simulink model "simulation1"  (R2018a)
settings: Solver=FixedStepAuto  StartTime=0.0  StopTime=300  FixedStep=0.1  RelTol=1e-3
values from neighbouring files (symbols this model uses):
  C_wn = C_w(:,4)    [Sim1.m]    (also in Sim3.m; Sim4_EKF.m; Sim4_Nolinear.m; Sim5_Nolinear.m)
  C_wx = C_w(:,2)    [Sim1.m]    (also in Sim3.m; Sim4_EKF.m; Sim4_Nolinear.m; Sim5_Nolinear.m)
  C_wy = C_w(:,3)    [Sim1.m]    (also in Sim3.m; Sim4_EKF.m; Sim4_Nolinear.m; Sim5_Nolinear.m)
  getPos = [0;0;1]    [Sim2.m]    (also in Sim3.m; Sim4_EKF.m; Sim4_Nolinear.m; Sim5_Nolinear.m)
  getVel = [0;1;0]    [Sim2.m]    (also in Sim3.m; Sim4_EKF.m; Sim4_Nolinear.m; Sim5_Nolinear.m)
  h = 0.1    [Sim1.m]    (also in Sim2.m; Sim3.m; Sim4_EKF.m; Sim4_Nolinear.m)
  Kd = 7*[2*M3(1)*Omega 0 0; 0 3*M3(2,2)*Omega 0; 0 0 20*M(3,3)*Omega]    [Sim2.m]    (also in Sim3.m; Sim4_EKF.m; Sim4_Nolinear.m; Sim5_Nolinear.m = 7*[30*M3(1)*Omega 0 0; 0 150*M3(2,2)*Omega 0; 0 0 30*M(3,3)*)
  Ki = 100*(omega/10)*[M3(1)*omega^2 0 0;0 0.05*M3(2,2)*omega^2 0; 0 0 M3(3,3)*omega^2 ]*2    [Sim2.m]    (also in Sim3.m; Sim4_EKF.m; Sim4_Nolinear.m; Sim5_Nolinear.m = 10*(omega/10)*[30*M3(1)*omega^2 0 0;0 150*M3(2,2)*omega^2 0;)
  Kp = 50*[6*M3(1)*omega^2 0 0;0 M3(2,2)*omega^2 0; 0 0 10*M3(3,3)*omega^2 ]    [Sim2.m]    (also in Sim3.m; Sim4_EKF.m; Sim4_Nolinear.m; Sim5_Nolinear.m = 5*[60*M3(1)*omega^2 0 0;0 800*M3(2,2)*omega^2 0; 0 0 30*M3(3)
  mu2_c = 0.001    [Sim1.m]    (also in Sim3.m; Sim4_EKF.m; Sim4_Nolinear.m; Sim5_Nolinear.m)
  mu2_w = 0.001    [Sim1.m]    (also in Sim3.m; Sim4_EKF.m; Sim4_Nolinear.m; Sim5_Nolinear.m)
  mu_w = 0.001    [Sim1.m]    (also in Sim3.m; Sim4_EKF.m; Sim4_Nolinear.m; Sim5_Nolinear.m)
  Omega = 2*damping*omega    [Sim2.m]    (also in Sim3.m; Sim4_EKF.m; Sim4_Nolinear.m = diag([omega_1,omega_2,omega_3]); Sim5_Nolinear.m = diag([omega_1,omega_2,omega_3]))
  omega = omegab/sqrt(1-2*damping^2+sqrt(4*damping^4-4*damping^2+2))    [Sim2.m]    (also in Sim3.m; Sim4_EKF.m; Sim4_Nolinear.m; Sim5_Nolinear.m)
  phi_c = -pi/2    (= -1.57079632679)    [Sim1.m]    (also in Sim3.m; Sim4_EKF.m; Sim4_Nolinear.m; Sim5_Nolinear.m)
  psi_r = C_w(:,1)    [Sim1.m]    (also in Sim3.m; Sim4_EKF.m; Sim4_Nolinear.m; Sim5_Nolinear.m)
  ref = [0;0;0]    [Sim2.m]    (also in Sim3.m; Sim4_EKF.m; Sim4_Nolinear.m; Sim5_Nolinear.m)
  V_mean = 0.5    [Sim1.m]    (also in Sim3.m; Sim4_EKF.m; Sim4_Nolinear.m; Sim5_Nolinear.m)
  W_gust = Ug    [Sim1.m]    (also in Sim3.m; Sim4_EKF.m; Sim4_Nolinear.m; Sim5_Nolinear.m)
  W_mean = 15    [Sim1.m]    (also in Sim3.m; Sim4_EKF.m; Sim4_Nolinear.m; Sim5_Nolinear.m)
undefined symbols (not defined in the file or in its folder): Hoerner, magnitude, vessel
libraries: simulink x3, marine_hydro x2, marine_gnc x1, simulink_extras x1
settings Model: Creator=jonbjor  LastModifiedBy=34275

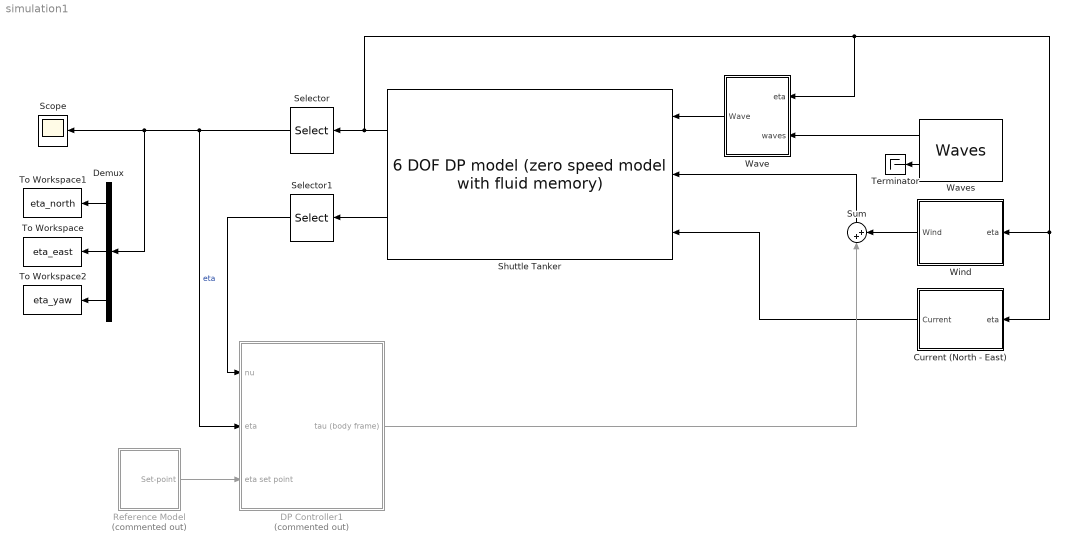
== system simulation1 ==
  Current (North - East) : Subsystem
  DP Controller1 : Subsystem  Commented=on
  Demux : Demux  Outputs=3
  Reference Model : Subsystem  Commented=on
  Scope : Scope
  Selector : Selector  InputPortWidth=6  IndexOptions=Index vector (dialog)  Indices=[1 2 6]  OutputSizes=1
  Selector1 : Selector  InputPortWidth=6  IndexOptions=Index vector (dialog)  Indices=[1 2 6]  OutputSizes=1
  Shuttle Tanker : marine_hydro/Hydro Library/6 DOF DP model  (zero speed model with fluid memory)  ABC=vesselABC  rho=1025  Axc=0.9*vessel.main.T*vessel.main.B  Ayc=0.9*vessel.main.T*vessel.main.Lpp  CX=1  CY_2D=Hoerner(vessel.main.B,vessel.main.T)  Bv=vessel.Bv  mask(6 DOF zero speed model){}
      link override "Integrator1 ": InitialCondition=nu0
      link override Integrator2: InitialCondition=eta0
      settings: SourceProductName=MSS Hydro
      mask Display:
      | image('shuttleTanker.jpg');
      | color('white'); port_label('output', 1, 'eta')
      | color('white'); port_label('output', 2, 'nu')
      | color('white'); port_label('input', 1, 'tau_wave')
      | color('white'); port_label('input', 2, 'tau')
      | color('white'); port_label('input', 3, 'nu_c')
  Sum : Sum  Inputs=|++
  Terminator : Terminator
  To Workspace : ToWorkspace  VariableName=eta_east  SaveFormat=Timeseries  SampleTime=-1
  To Workspace1 : ToWorkspace  VariableName=eta_north  SaveFormat=Timeseries  SampleTime=-1
  To Workspace2 : ToWorkspace  VariableName=eta_yaw  SaveFormat=Timeseries  SampleTime=-1
  Wave : Subsystem  mask{waveforces=on}
      mask prompts: waveforces "Waveforces enabled"
  Waves : marine_gnc/Environment/Waves/Waves  spectrum_type=ITTC  disp_flag=on  plot_spectrum=off  plot_realization=off  hs=2.5  omega_peak=pi/4.5  psi_mean=5*pi/8  gamma=-1  spread=2  depth=inf  nfreq=20  ndir=10  energylim=0.005  freq_cutoff=3  dir_cutoff=0  rand_seed=123  rand_freq=on  rand_dir=on  Zeta_a=0  Omega=0  Phase=0  Wavenum=0  Psi=0
      settings: SourceProductName=MSS GNC
  Wind : Subsystem
  wires:
  Shuttle Tanker/2 -> Selector1/1
  Reference Model/1(Set-point) -> DP Controller1/3(eta set point)
  Shuttle Tanker/1 -> Selector/1, Current (North - East)/1(eta), Wind/1(eta), Wave/1(eta)
  Wave/1(Wave) -> Shuttle Tanker/1
  Waves/1 -> Wave/2(waves)
  Waves/2 -> Terminator/1
  Selector1/1 -> DP Controller1/1(nu)
  Wind/1(Wind) -> Sum/2
  Sum/1 -> Shuttle Tanker/2
  Selector/1 -> DP Controller1/2(eta), Demux/1, Scope/1  "eta"
  Current (North - East)/1(Current) -> Shuttle Tanker/3
  DP Controller1/1(tau (body frame)) -> Sum/1
  Demux/3 -> To Workspace2/1
  Demux/1 -> To Workspace1/1
  Demux/2 -> To Workspace/1

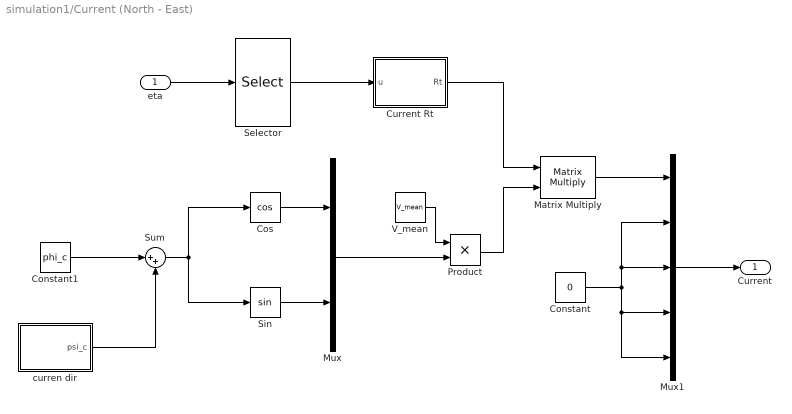
== system simulation1/Current (North - East) ==
  eta : Inport
  Constant : Constant  Value=0
  Constant1 : Constant  Value=phi_c
  Cos : Trigonometry  Operator=cos
  Current Rt : MATLAB Function  TreatAsAtomicUnit=on
  Matrix Multiply : Product  Multiplication=Matrix(*)
  Mux : Mux  Inputs=2
  Mux1 : Mux  Inputs=5
  Product : Product
  Selector : Selector  InputPortWidth=6  IndexOptions=Index vector (dialog)  Indices=[6]  OutputSizes=1
  Sin : Trigonometry
  Sum : Sum  Inputs=|++
  V_mean : Constant  Value=V_mean
  curren dir : Subsystem
  Current : Outport
  wires:
  V_mean/1 -> Product/1
  Mux1/1 -> Current/1
  Cos/1 -> Mux/1
  Mux/1 -> Product/2
  Sin/1 -> Mux/2
  Constant/1 -> Mux1/5, Mux1/4, Mux1/3, Mux1/2
  Constant1/1 -> Sum/1
  curren dir/1("psi_c ") -> Sum/2
  Sum/1 -> Sin/1, Cos/1
  eta/1 -> Selector/1
  Selector/1 -> Current Rt/1(u)
  Current Rt/1(Rt) -> Matrix Multiply/1
  Product/1 -> Matrix Multiply/2
  Matrix Multiply/1 -> Mux1/1

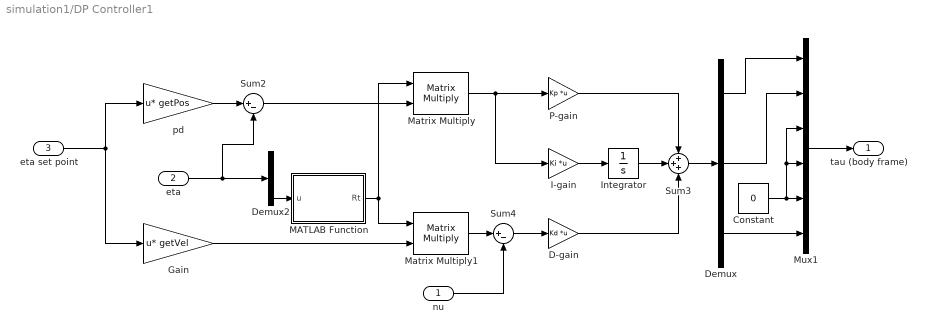
== system simulation1/DP Controller1 ==
  nu : Inport
  eta : Inport  Port=2
  eta set point : Inport  Port=3
  Constant : Constant  Value=0
  D-gain : Gain  Gain=Kd  Multiplication=Matrix(K*u)
  Demux : Demux  Outputs=3
  Demux2 : Demux  Outputs=3
  Gain : Gain  Gain=getVel  Multiplication=Matrix(u*K)
  I-gain : Gain  Gain=Ki  Multiplication=Matrix(K*u)
  Integrator : Integrator
  MATLAB Function : MATLAB Function  TreatAsAtomicUnit=on
  Matrix Multiply : Product  Multiplication=Matrix(*)
  Matrix Multiply1 : Product  Multiplication=Matrix(*)
  Mux1 : Mux  Inputs=6
  P-gain : Gain  Gain=Kp  Multiplication=Matrix(K*u)
  Sum2 : Sum  Inputs=|+-
  Sum3 : Sum  Inputs=+++
  Sum4 : Sum  Inputs=|+-
  pd : Gain  Gain=getPos  Multiplication=Matrix(u*K)
  tau (body frame) : Outport
  wires:
  Demux2/3 -> MATLAB Function/1(u)
  pd/1 -> Sum2/1
  Matrix Multiply/1 -> I-gain/1, P-gain/1
  Mux1/1 -> tau (body frame)/1
  Demux/3 -> Mux1/6
  Integrator/1 -> Sum3/2
  Demux/2 -> Mux1/2
  P-gain/1 -> Sum3/1
  nu/1 -> Sum4/2
  Sum2/1 -> Matrix Multiply/2
  D-gain/1 -> Sum3/3
  MATLAB Function/1(Rt) -> Matrix Multiply1/1, Matrix Multiply/1
  Demux/1 -> Mux1/1
  Matrix Multiply1/1 -> Sum4/1
  Constant/1 -> Mux1/4, Mux1/3, Mux1/5
  eta set point/1 -> Gain/1, pd/1
  Gain/1 -> Matrix Multiply1/2
  Sum3/1 -> Demux/1
  Sum4/1 -> D-gain/1
  I-gain/1 -> Integrator/1
  eta/1 -> Demux2/1, Sum2/2

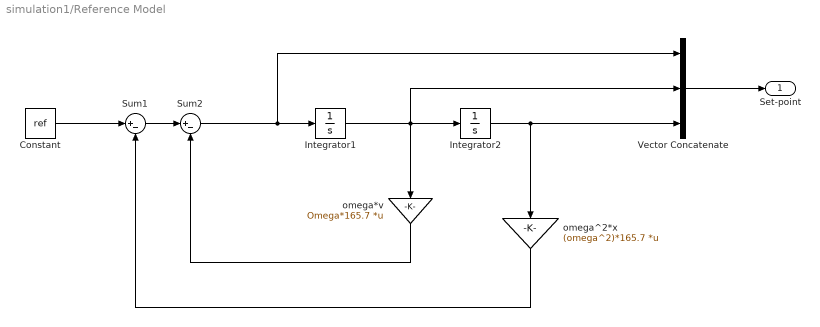
== system simulation1/Reference Model ==
  Constant : Constant  Value=ref
  Integrator1 : Integrator
  Integrator2 : Integrator
  Sum1 : Sum  Inputs=|+-
  Sum2 : Sum  Inputs=|+-
  Vector Concatenate : Concatenate  NumInputs=3  Mode=Multidimensional array  ConcatenateDimension=2
  omega*v : Gain  Gain=Omega*165.7  Multiplication=Matrix(K*u)
  omega^2*x : Gain  Gain=(omega^2)*165.7  Multiplication=Matrix(K*u)
  Set-point : Outport
  wires:
  omega^2*x/1 -> Sum1/2
  Integrator2/1 -> Vector Concatenate/3, omega^2*x/1
  Sum1/1 -> Sum2/1
  Integrator1/1 -> Vector Concatenate/2, omega*v/1, Integrator2/1
  Constant/1 -> Sum1/1
  Sum2/1 -> Vector Concatenate/1, Integrator1/1
  omega*v/1 -> Sum2/2
  Vector Concatenate/1 -> Set-point/1

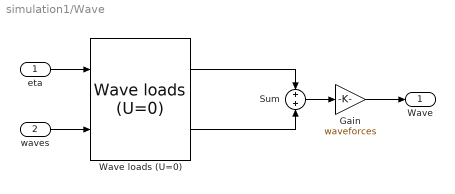
== system simulation1/Wave ==
  eta : Inport
  waves : Inport  Port=2
  Gain : Gain  Gain=waveforces
  Sum : Sum
  Wave loads (U=0) : marine_hydro/Hydro Library/Wave loads (U=0)
      settings: SourceProductName=MSS Hydro
  Wave : Outport
  wires:
  eta/1 -> Wave loads (U=0)/1
  waves/1 -> Wave loads (U=0)/2
  Sum/1 -> Gain/1
  Wave loads (U=0)/1 -> Sum/1
  Wave loads (U=0)/2 -> Sum/2
  Gain/1 -> Wave/1

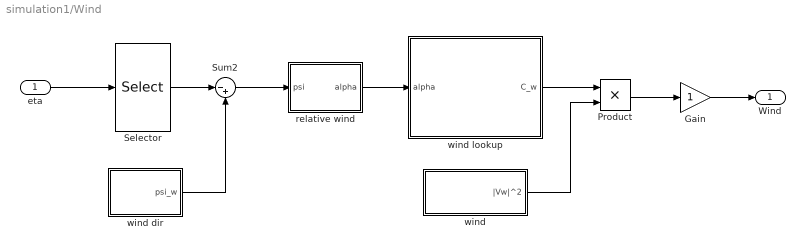
== system simulation1/Wind ==
  eta : Inport
  Gain : Gain
  Product : Product
  Selector : Selector  InputPortWidth=6  IndexOptions=Index vector (dialog)  Indices=[6]  OutputSizes=1
  Sum2 : Sum  Inputs=|-+
  relative wind : MATLAB Function  TreatAsAtomicUnit=on
  wind : Subsystem
  wind dir : Subsystem
  wind lookup : Subsystem
  Wind : Outport
  wires:
  wind lookup/1(C_w) -> Product/1
  relative wind/1(alpha) -> wind lookup/1(alpha)
  Sum2/1 -> relative wind/1(psi)
  wind dir/1(psi_w) -> Sum2/2
  wind/1(|Vw|^2) -> Product/2
  Product/1 -> Gain/1
  eta/1 -> Selector/1
  Selector/1 -> Sum2/1
  Gain/1 -> Wind/1

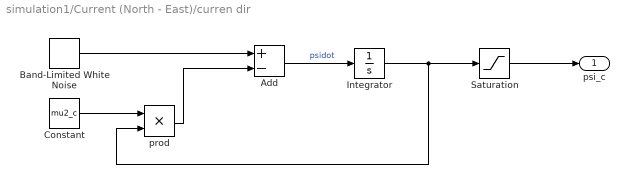
== system simulation1/Current (North - East)/curren dir ==
  Add : Sum  Inputs=+-
  Band-Limited White Noise : simulink/Sources/Band-Limited White Noise  Cov=w  Ts=h  seed=[23341]
  Constant : Constant  Value=mu2_c
  Integrator : Integrator
  Saturation : Saturate  UpperLimit=5*pi/180  LowerLimit=5*pi/180
  prod : Product  Inputs=**
  "psi_c " : Outport
  wires:
  Add/1 -> Integrator/1  "psidot"
  prod/1 -> Add/2
  Band-Limited White Noise/1 -> Add/1
  Constant/1 -> prod/1
  Integrator/1 -> Saturation/1, prod/2
  Saturation/1 -> "psi_c "/1

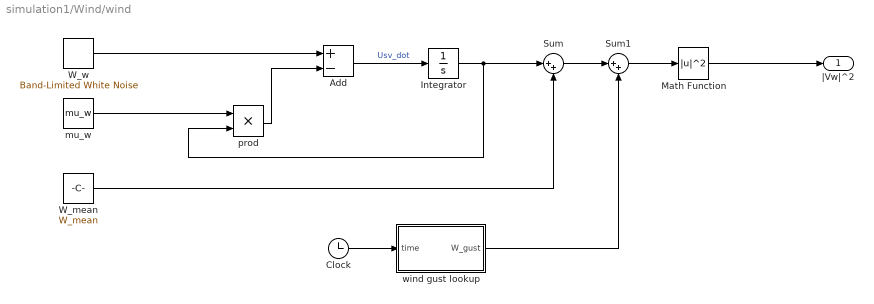
== system simulation1/Wind/wind ==
  Add : Sum  Inputs=+-
  Clock : Clock
  Integrator : Integrator
  Math Function : Math  Operator=magnitude^2  SaturateOnIntegerOverflow=on
  Sum : Sum  Inputs=|++
  Sum1 : Sum  Inputs=|++
  "W_mean " : Constant  Value=W_mean
  W_w : simulink/Sources/Band-Limited White Noise  Cov=w  Ts=0.1  seed=[23341]
  mu_w : Constant  Value=mu_w
  prod : Product  Inputs=**
  wind gust lookup : Subsystem
  |Vw|^2 : Outport
  wires:
  Add/1 -> Integrator/1  "Usv_dot"
  prod/1 -> Add/2
  Math Function/1 -> |Vw|^2/1
  "W_mean "/1 -> Sum/2
  W_w/1 -> Add/1
  mu_w/1 -> prod/1
  Integrator/1 -> Sum/1, prod/2
  Sum/1 -> Sum1/1
  Sum1/1 -> Math Function/1
  wind gust lookup/1(W_gust) -> Sum1/2
  Clock/1 -> wind gust lookup/1(time)

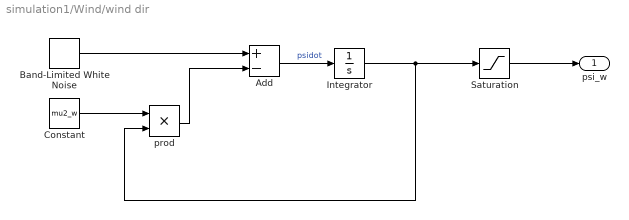
== system simulation1/Wind/wind dir ==
  Add : Sum  Inputs=+-
  Band-Limited White Noise : simulink/Sources/Band-Limited White Noise  Cov=w  Ts=h  seed=[23341]
  Constant : Constant  Value=mu2_w
  Integrator : Integrator
  Saturation : Saturate  UpperLimit=5*pi/180  LowerLimit=5*pi/180
  prod : Product  Inputs=**
  psi_w : Outport
  wires:
  Add/1 -> Integrator/1  "psidot"
  prod/1 -> Add/2
  Band-Limited White Noise/1 -> Add/1
  Constant/1 -> prod/1
  Integrator/1 -> Saturation/1, prod/2
  Saturation/1 -> psi_w/1

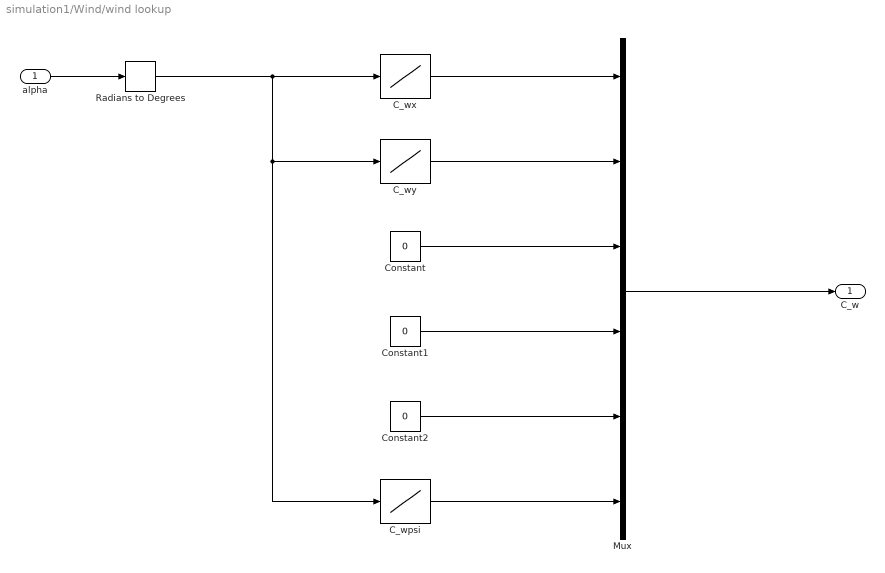
== system simulation1/Wind/wind lookup ==
  alpha : Inport
  C_wpsi : Lookup_n-D  NumberOfTableDimensions=1  BreakpointsForDimension1=psi_r  Table=C_wn  InternalRulePriority=Speed  RndMeth=Simplest  InputSameDT=on
  C_wx : Lookup_n-D  NumberOfTableDimensions=1  BreakpointsForDimension1=psi_r  Table=C_wx  InternalRulePriority=Speed  RndMeth=Simplest  InputSameDT=on
  C_wy : Lookup_n-D  NumberOfTableDimensions=1  BreakpointsForDimension1=psi_r  Table=C_wy  InternalRulePriority=Speed  RndMeth=Simplest  InputSameDT=on
  Constant : Constant  Value=0
  Constant1 : Constant  Value=0
  Constant2 : Constant  Value=0
  Mux : Mux  Inputs=6
  Radians to Degrees : simulink_extras/Transformations/Radians to Degrees
  C_w : Outport
  wires:
  C_wx/1 -> Mux/1
  C_wy/1 -> Mux/2
  Constant/1 -> Mux/3
  Constant1/1 -> Mux/4
  Constant2/1 -> Mux/5
  C_wpsi/1 -> Mux/6
  Mux/1 -> C_w/1
  alpha/1 -> Radians to Degrees/1
  Radians to Degrees/1 -> C_wpsi/1, C_wy/1, C_wx/1

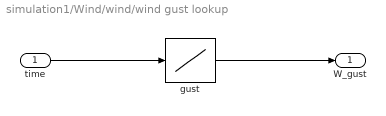
== system simulation1/Wind/wind/wind gust lookup ==
  time : Inport
  gust : Lookup_n-D  NumberOfTableDimensions=1  BreakpointsForDimension1=t  Table=W_gust  InternalRulePriority=Speed  RndMeth=Simplest  InputSameDT=on
  W_gust : Outport
  wires:
  gust/1 -> W_gust/1
  time/1 -> gust/1

== matlab function simulation1/Current (North - East)/Current Rt ==
  data: u input; Rt output
function Rt = fcn(u)

R=[cos(u) -sin(u); sin(u) cos(u)];
Rt=transpose(R);

end

== matlab function simulation1/Wind/relative wind ==
  data: psi input; alpha output
function alpha = psi2alpha(psi)

alph = pi-psi;

if alph < 0
    alph = alph+2*pi;
end

alpha = alph;

== matlab function simulation1/DP Controller1/MATLAB Function ==
  data: u input; Rt output
function Rt = fcn(u)

R=[cos(u) -sin(u) 0; sin(u) cos(u) 0; 0 0 1];
Rt=transpose(R);

end
